simulink library "lib_ForwardKinematicsMacroRobot"  (R2023b)
settings: Solver=VariableStepAuto  StartTime=0.0  StopTime=10.0  RelTol=1e-3
undefined symbols (not defined in the file or in its folder): robotParameters, robotStateStruct
settings Model: Creator=murali  LastModifiedBy=Murali Karnam
settings SolverCC: AlgebraicLoopSolver=TrustRegion
settings DataIOCC: ReturnWorkspaceOutputs=off
settings DebuggingCC: UnconnectedInputMsg=warning  UnconnectedOutputMsg=warning  UnconnectedLineMsg=warning  ArithmeticOperatorsInVariantConditions=warning
settings ModelReferenceCC: EnableRefExpFcnMdlSchedulingChecks=on
settings SFSimCC: SimUseLocalCustomCode=off  CustomCodeUndefinedFunction=UseInterfaceOnly
settings RTWCC: RTWUseLocalCustomCode=off

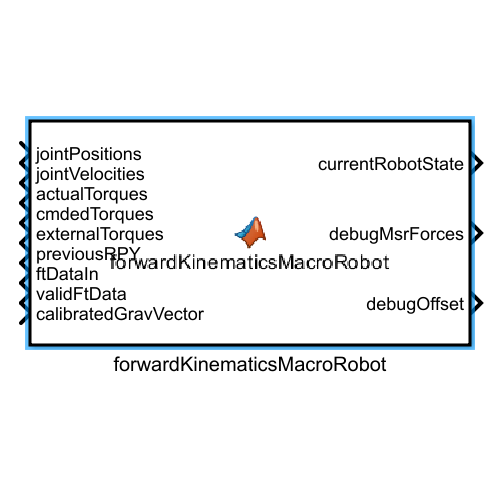
[thumbnail: Simulink's stored preview of the top-level diagram]
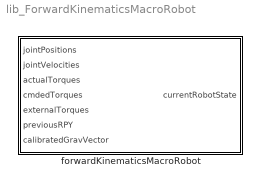
== system lib_ForwardKinematicsMacroRobot ==
  forwardKinematicsMacroRobot : MATLAB Function  TreatAsAtomicUnit=on

== matlab function lib_ForwardKinematicsMacroRobot/forwardKinematicsMacroRobot ==
  data: jointPositions input double size=[nJointsKuka,1]; jointVelocities input double size=[nJointsKuka,1]; actualTorques input double size=[nJointsKuka,1]; cmdedTorques input double size=[nJointsKuka,1]; externalTorques input double size=[nJointsKuka,1]; currentRobotState output Bus: RobotState size=1; robotParameters parameter; previousRPY input double size=[3,1]; robotStateStruct parameter Bus: RobotState; calibratedGravVector input double size=[3 1]
%#codegen
function currentRobotState  = forwardKinematicsMacroRobot(jointPositions, jointVelocities, actualTorques, cmdedTorques, externalTorques, robotParameters, previousRPY, robotStateStruct, calibratedGravVector)

% This just calls the function fun_ForwardKinematicsMacroRobot.m, which has
% the actual code to find the robotstate.

currentRobotState = fun_ForwardKinematicsMacroRobot(jointPositions, jointVelocities, actualTorques, cmdedTorques, externalTorques, robotParameters, robotStateStruct, previousRPY, calibratedGravVector);

end
